simulink model "SeriesWoundDCMotor_model"  (R2023a)
settings: Solver=VariableStepAuto  StartTime=0.0  StopTime=10.0  RelTol=1e-3
values from neighbouring files (symbols this model uses):
  C_M = 1.3    [Constants.m]
  C_W = 3.15    [Constants.m]
  J_mot = 7*10^-6    (= 7e-06)    [Constants.m]
  L_a = 0.0015    [Constants.m]
  L_fw = 0.013    [Constants.m]
  R_a = 8    [Constants.m]
undefined symbols (not defined in the file or in its folder): beta
settings Model: Creator=dmitr  LastModifiedBy=dmitr

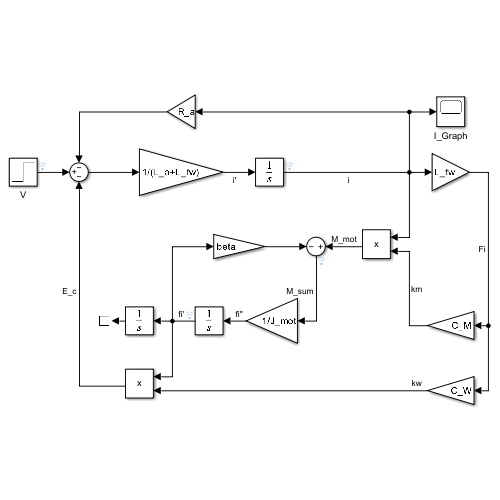
[thumbnail: Simulink's stored preview of the top-level diagram]
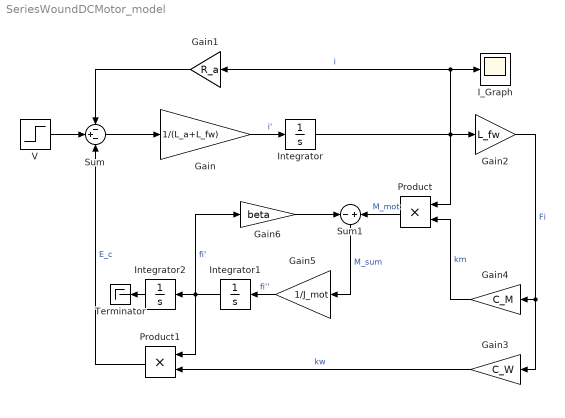
== system SeriesWoundDCMotor_model ==
  Gain : Gain  Gain=1/(L_a+L_fw)
  Gain1 : Gain  Gain=R_a
  Gain2 : Gain  Gain=L_fw
  Gain3 : Gain  Gain=C_W
  Gain4 : Gain  Gain=C_M
  Gain5 : Gain  Gain=1/J_mot
  Gain6 : Gain  Gain=beta
  I_Graph : Scope
  Integrator : Integrator
  Integrator1 : Integrator
  Integrator2 : Integrator
  Product : Product
  Product1 : Product
  Sum : Sum  Inputs=-+-
  Sum1 : Sum  Inputs=-|+
  Terminator : Terminator
  V : Step  Time=0  After=10  SampleTime=0
  wires:
  V/1 -> Sum/2
  Sum/1 -> Gain/1
  Gain/1 -> Integrator/1  "i'"
  Integrator/1 -> Gain1/1, I_Graph/1, Gain2/1, Product/1  "i"
  Gain1/1 -> Sum/1
  Gain2/1 -> Gain3/1, Gain4/1  "Fi"
  Gain4/1 -> Product/2  "km"
  Gain5/1 -> Integrator1/1  "fi''"
  Integrator1/1 -> Gain6/1, Product1/1, Integrator2/1  "fi'"
  Gain3/1 -> Product1/2  "kw"
  Product1/1 -> Sum/3  "E_c"
  Integrator2/1 -> Terminator/1
  Product/1 -> Sum1/2  "M_mot"
  Sum1/1 -> Gain5/1  "M_sum"
  Gain6/1 -> Sum1/1
